simulink model "Klausur_fi_wi_ma"  (R2021b)
settings: Solver=FixedStepAuto  StartTime=0.0  StopTime=753.0  FixedStep=0,5  RelTol=1e-3
values from neighbouring files (symbols this model uses):
  A = 2.5    [untitled.m]
  cw = 0.4    [untitled.m]
  d = 0.6    [untitled.m]
  g = 9.81    [untitled.m]
  Height = load("Hoehe.txt")    [untitled.m]
  i1 = 12.5    [untitled.m]
  i2 = 5    [untitled.m]
  m = 2000    [untitled.m]
  max_torque = xlsread("Motorkennlinie.xlsx","C16:O16")    [untitled.m]
  p = 1.2    [untitled.m]
  RPM = out.RPM    [untitled.m]
  Time = load("Zeit.txt")    [untitled.m]
  Velocity = load("Geschwindigkeit.txt")    [untitled.m]
undefined symbols (not defined in the file or in its folder): f_roll, J, n
settings Model: Creator=under  LastModifiedBy=user

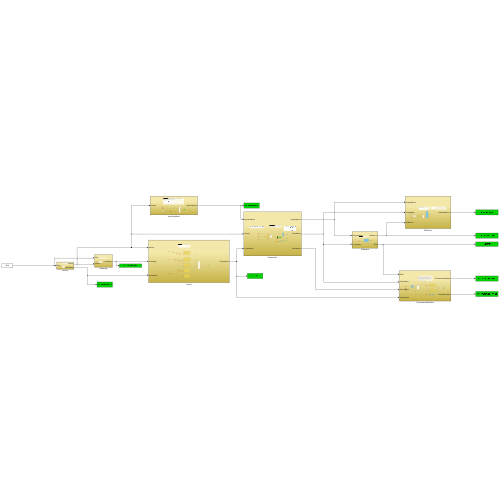
[thumbnail: Simulink's stored preview of the top-level diagram]
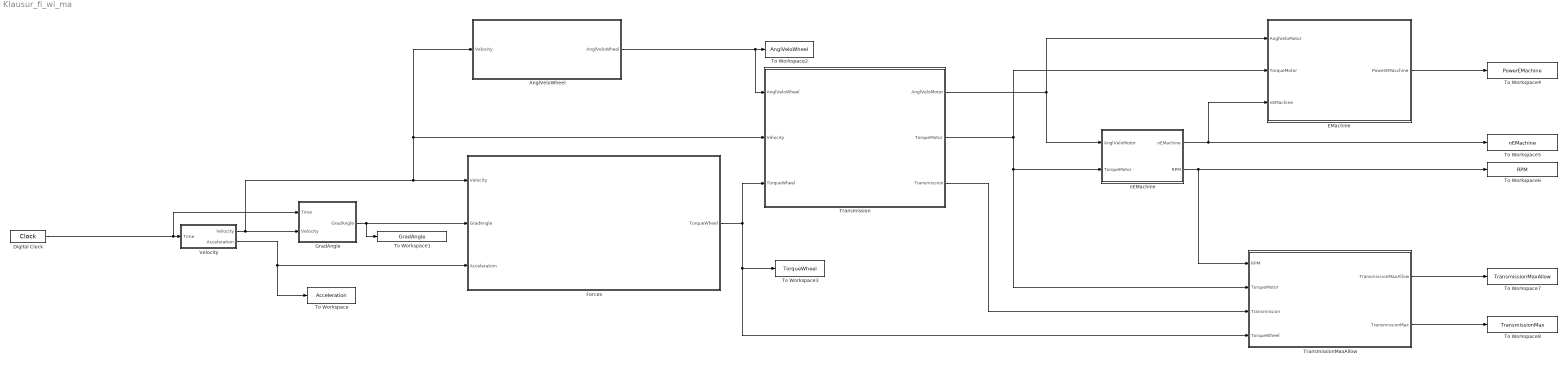
== system Klausur_fi_wi_ma ==
  AnglVeloWheel : Subsystem
  Digital Clock : DigitalClock
  EMachine : Subsystem
  Forces : Subsystem
  GradAngle : Subsystem
  To Workspace : ToWorkspace  VariableName=Acceleration  SaveFormat=Timeseries  SampleTime=-1
  To Workspace1 : ToWorkspace  VariableName=GradAngle  SaveFormat=Timeseries  SampleTime=-1
  To Workspace2 : ToWorkspace  VariableName=AnglVeloWheel  SaveFormat=Timeseries  SampleTime=-1
  To Workspace3 : ToWorkspace  VariableName=TorqueWheel  SaveFormat=Timeseries  SampleTime=-1
  To Workspace4 : ToWorkspace  VariableName=PowerEMachine  SaveFormat=Timeseries  SampleTime=-1
  To Workspace5 : ToWorkspace  VariableName=nEMachine  SaveFormat=Timeseries  SampleTime=-1
  To Workspace6 : ToWorkspace  VariableName=RPM  SaveFormat=Timeseries  SampleTime=-1
  To Workspace7 : ToWorkspace  VariableName=TransmissionMaxAllow  SaveFormat=Timeseries  SampleTime=-1
  To Workspace8 : ToWorkspace  VariableName=TransmissionMax  SaveFormat=Timeseries  SampleTime=-1
  Transmission : Subsystem
  TransmissionMaxAllow : Subsystem
  Velocity : Subsystem
  nEMachine : Subsystem
  wires:
  Transmission/2(TorqueMotor) -> TransmissionMaxAllow/2(TorqueMotor), nEMachine/2(TorqueMotor), EMachine/2(TorqueMotor)
  GradAngle/1(GradAngle) -> To Workspace1/1, Forces/2(GradAngle)
  Forces/1(TorqueWheel) -> TransmissionMaxAllow/4(TorqueWheel), To Workspace3/1, Transmission/3(TorqueWheel)
  Velocity/1(Velocity) -> AnglVeloWheel/1(Velocity), Transmission/2(Velocity), Forces/1(Velocity), GradAngle/2(Velocity)
  Digital Clock/1 -> GradAngle/1(Time), Velocity/1(Time)
  Transmission/1(AnglVeloMotor) -> EMachine/1(AnglVeloMotor), nEMachine/1(AnglVeloMotor)
  Velocity/2(Acceleration) -> To Workspace/1, Forces/3(Acceleration)
  AnglVeloWheel/1(AnglVeloWheel) -> Transmission/1(AnglVeloWheel), To Workspace2/1
  nEMachine/1(nEMachine) -> EMachine/3(nEMachine), To Workspace5/1
  EMachine/1(PowerEMaschine) -> To Workspace4/1
  nEMachine/2(RPM) -> TransmissionMaxAllow/1(RPM), To Workspace6/1
  Transmission/3(Transmission) -> TransmissionMaxAllow/3(Transmission)
  TransmissionMaxAllow/1(TransmissionMaxAllow) -> To Workspace7/1
  TransmissionMaxAllow/2(TransmissionMax) -> To Workspace8/1

== system Klausur_fi_wi_ma/AnglVeloWheel ==
  note: AnglVeloWheel
      | In diesem Subsystem wird die Geschwindigkeit und der Reifenradius dividiert, so wird die Winkelgeschwindigkeit ausgerechnet.
  Velocity : Inport
  Divide : Product  Inputs=*/
  WheelDiam : Constant  Value=d
  dToR : Gain  Gain=1/2
  AnglVeloWheel : Outport
  wires:
  dToR/1 -> Divide/2
  Velocity/1 -> Divide/1
  Divide/1 -> AnglVeloWheel/1
  WheelDiam/1 -> dToR/1

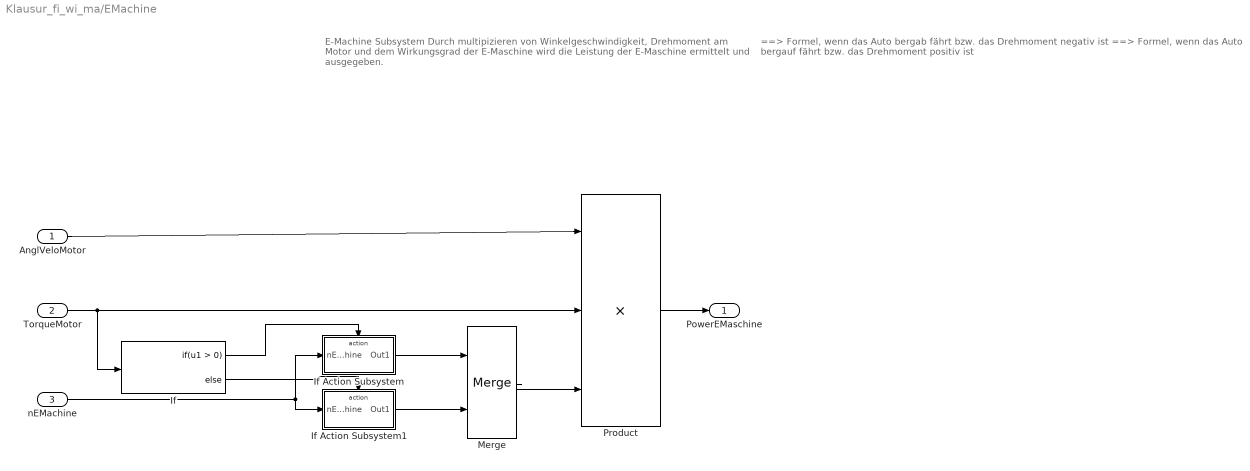
== system Klausur_fi_wi_ma/EMachine ==
  note: ==> Formel, wenn das Auto bergab fährt bzw. das Drehmoment negativ ist
      | ==> Formel, wenn das Auto bergauf fährt bzw. das Drehmoment positiv ist
  note: E-Machine Subsystem
      | Durch multipizieren von Winkelgeschwindigkeit, Drehmoment am Motor und dem Wirkungsgrad der E-Maschine wird die Leistung der E-Maschine ermittelt und ausgegeben.
  AnglVeloMotor : Inport
  TorqueMotor : Inport  Port=2
  nEMachine : Inport  Port=3
  If : If
  If Action Subsystem : Subsystem  TreatAsAtomicUnit=on
  If Action Subsystem1 : Subsystem  TreatAsAtomicUnit=on
  Merge : Merge
  Product : Product  Inputs=3
  PowerEMaschine : Outport
  wires:
  TorqueMotor/1 -> If/1, Product/2
  nEMachine/1 -> If Action Subsystem1/1(nEMachine), If Action Subsystem/1(nEMachine)
  If/2 -> If Action Subsystem1/Action
  If/1 -> If Action Subsystem/Action
  Product/1 -> PowerEMaschine/1
  Merge/1 -> Product/3
  If Action Subsystem/1(Out1) -> Merge/1
  If Action Subsystem1/1(Out1) -> Merge/2
  AnglVeloMotor/1 -> Product/1

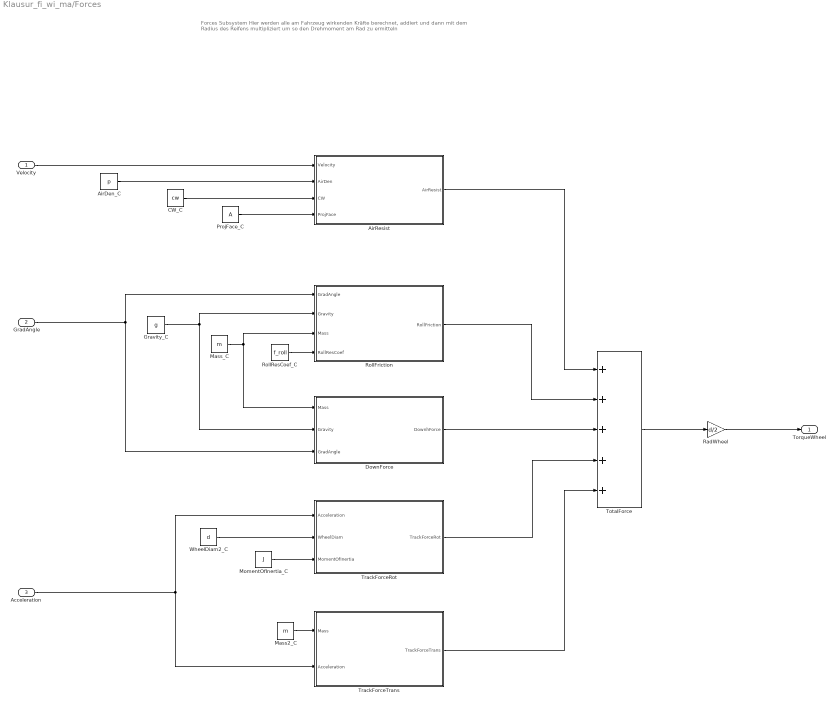
== system Klausur_fi_wi_ma/Forces ==
  note: Forces Subsystem
      | Hier werden alle am Fahrzeug wirkenden Kräfte berechnet, addiert und dann mit dem Radius des Reifens multipliziert um so den Drehmoment am Rad zu ermitteln
  Velocity : Inport
  GradAngle : Inport  Port=2
  Acceleration : Inport  Port=3
  AirDen_C : Constant  Value=p
  AirResist : Subsystem
  CW_C : Constant  Value=cw
  DownForce : Subsystem
  Gravity_C : Constant  Value=g
  Mass2_C : Constant  Value=m
  Mass_C : Constant  Value=m
  MomentOfInertia_C : Constant  Value=J
  ProjFace_C : Constant  Value=A
  RadWheel : Gain  Gain=d/2
  RollFriction : Subsystem
  RollResCoef_C : Constant  Value=f_roll
  TotalForce : Sum  Inputs=+++++
  TrackForceRot : Subsystem
  TrackForceTrans : Subsystem
  WheelDiam2_C : Constant  Value=d
  TorqueWheel : Outport
  wires:
  GradAngle/1 -> DownForce/3(GradAngle), RollFriction/1(GradAngle)
  Gravity_C/1 -> DownForce/2(Gravity), RollFriction/2(Gravity)
  RollResCoef_C/1 -> RollFriction/4(RollResCoef)
  Mass_C/1 -> DownForce/1(Mass), RollFriction/3(Mass)
  TotalForce/1 -> RadWheel/1
  Acceleration/1 -> TrackForceTrans/2(Acceleration), TrackForceRot/1(Acceleration)
  TrackForceRot/1(TrackForceRot) -> TotalForce/4
  TrackForceTrans/1(TrackForceTrans) -> TotalForce/5
  WheelDiam2_C/1 -> TrackForceRot/2(WheelDiam)
  MomentOfInertia_C/1 -> TrackForceRot/3(MomentOfInertia)
  Mass2_C/1 -> TrackForceTrans/1(Mass)
  RadWheel/1 -> TorqueWheel/1
  AirResist/1(AirResist) -> TotalForce/1
  Velocity/1 -> AirResist/1(Velocity)
  ProjFace_C/1 -> AirResist/4(ProjFace)
  CW_C/1 -> AirResist/3(CW)
  AirDen_C/1 -> AirResist/2(AirDen)
  RollFriction/1(RollFriction) -> TotalForce/2
  DownForce/1(DownhForce) -> TotalForce/3

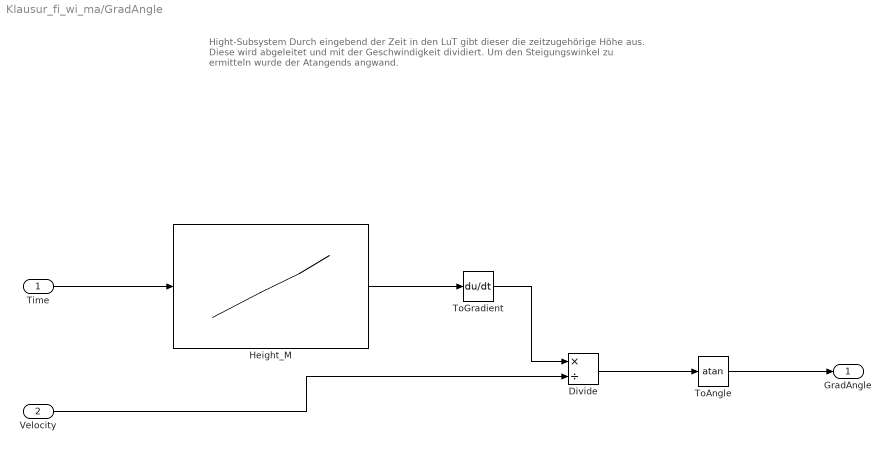
== system Klausur_fi_wi_ma/GradAngle ==
  note: Hight-Subsystem
      | Durch eingebend der Zeit in den LuT gibt dieser die zeitzugehörige Höhe aus. Diese wird abgeleitet und mit der Geschwindigkeit dividiert. Um den Steigungswinkel zu ermitteln wurde der Atangends angwand.
  Time : Inport
  Velocity : Inport  Port=2
  Divide : Product  Inputs=*/
  Height_M : Lookup_n-D  NumberOfTableDimensions=1  BreakpointsForDimension1=Time  Table=Height  InternalRulePriority=Speed  RndMeth=Simplest  InputSameDT=on
  ToAngle : Trigonometry  Operator=atan
  ToGradient : Derivative
  GradAngle : Outport
  wires:
  ToAngle/1 -> GradAngle/1
  Divide/1 -> ToAngle/1
  Velocity/1 -> Divide/2
  ToGradient/1 -> Divide/1
  Height_M/1 -> ToGradient/1
  Time/1 -> Height_M/1

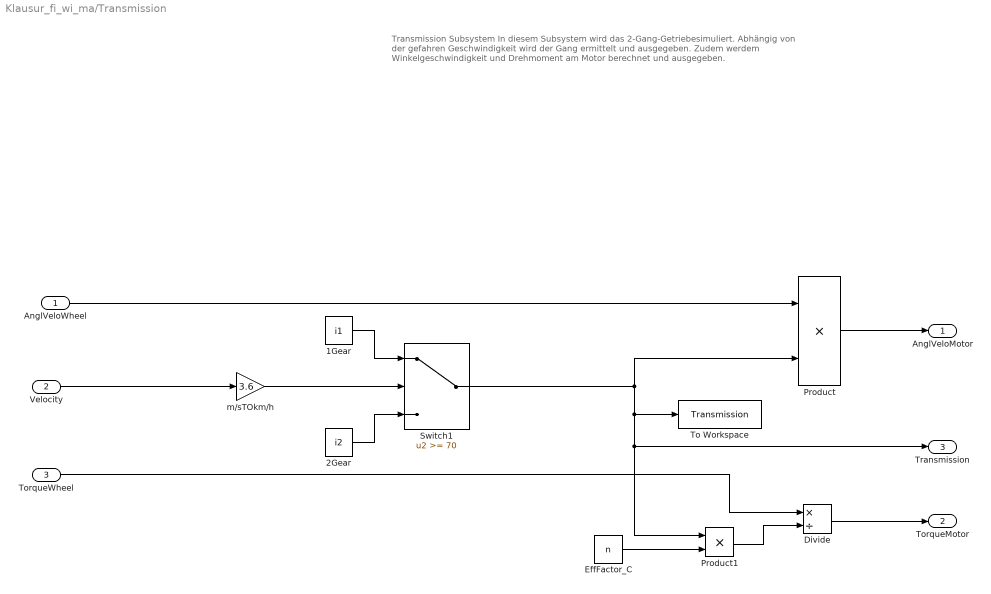
== system Klausur_fi_wi_ma/Transmission ==
  note: Transmission Subsystem
      | In diesem Subsystem wird das 2-Gang-Getriebesimuliert. Abhängig von der gefahren Geschwindigkeit wird der Gang ermittelt und ausgegeben.
      | Zudem werdem Winkelgeschwindigkeit und Drehmoment am Motor berechnet und ausgegeben.
  AnglVeloWheel : Inport
  Velocity : Inport  Port=2
  TorqueWheel : Inport  Port=3
  1Gear : Constant  Value=i1
  2Gear : Constant  Value=i2
  Divide : Product  Inputs=*/
  EffFactor_C : Constant  Value=n
  Product : Product
  Product1 : Product
  Switch1 : Switch  Threshold=70
  To Workspace : ToWorkspace  VariableName=Transmission  SaveFormat=Timeseries  SampleTime=-1
  "m/sTOkm/h  " : Gain  Gain=3.6
  AnglVeloMotor : Outport
  TorqueMotor : Outport  Port=2
  Transmission : Outport  Port=3
  wires:
  "m/sTOkm/h  "/1 -> Switch1/2
  Switch1/1 -> Transmission/1, Product1/1, To Workspace/1, Product/2
  Product/1 -> AnglVeloMotor/1
  EffFactor_C/1 -> Product1/2
  Product1/1 -> Divide/2
  TorqueWheel/1 -> Divide/1
  Divide/1 -> TorqueMotor/1
  Velocity/1 -> "m/sTOkm/h  "/1
  AnglVeloWheel/1 -> Product/1
  1Gear/1 -> Switch1/1
  2Gear/1 -> Switch1/3

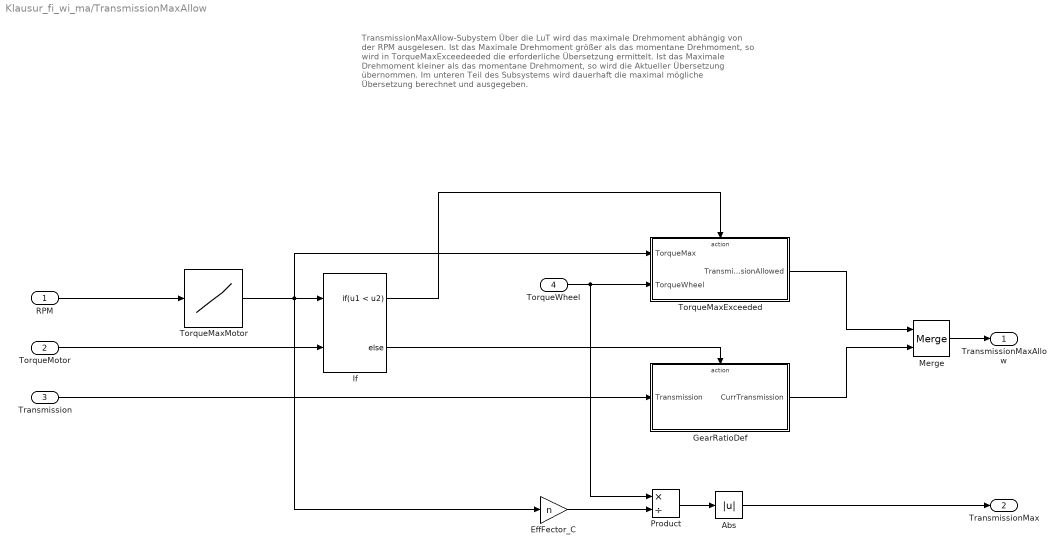
== system Klausur_fi_wi_ma/TransmissionMaxAllow ==
  note: TransmissionMaxAllow-Subystem
      | Über die LuT wird das maximale Drehmoment abhängig von der RPM ausgelesen. Ist das Maximale Drehmoment größer als das momentane Drehmoment, so wird in TorqueMaxExceedeeded die erforderliche Übersetzung ermittelt. Ist das Maximale Drehmoment kleiner als das momentane Drehmoment, so wird die Aktueller Übersetzung übernommen.
      | Im unteren Teil des Subsystems wird dauerhaft die maximal mögliche Übersetzung berechnet und ausgegeben.
  RPM : Inport
  TorqueMotor : Inport  Port=2
  Transmission : Inport  Port=3
  TorqueWheel : Inport  Port=4
  Abs : Abs
  EffFector_C : Gain  Gain=n
  GearRatioDef : Subsystem  TreatAsAtomicUnit=on
  If : If  NumInputs=2  IfExpression=u1 < u2
  Merge : Merge
  Product : Product  Inputs=*/
  TorqueMaxExceeded : Subsystem  TreatAsAtomicUnit=on
  TorqueMaxMotor : Lookup_n-D  NumberOfTableDimensions=1  BreakpointsForDimension1=RPM  Table=max_torque  InternalRulePriority=Speed  RndMeth=Simplest  InputSameDT=on
  TransmissionMaxAllow : Outport
  TransmissionMax : Outport  Port=2
  wires:
  Abs/1 -> TransmissionMax/1
  TorqueMaxMotor/1 -> EffFector_C/1, If/1, TorqueMaxExceeded/1(TorqueMax)
  If/1 -> TorqueMaxExceeded/Action
  TorqueWheel/1 -> Product/1, TorqueMaxExceeded/2(TorqueWheel)
  EffFector_C/1 -> Product/2
  Product/1 -> Abs/1
  TorqueMaxExceeded/1(TransmissionAllowed) -> Merge/1
  GearRatioDef/1(CurrTransmission) -> Merge/2
  RPM/1 -> TorqueMaxMotor/1
  TorqueMotor/1 -> If/2
  If/2 -> GearRatioDef/Action
  Transmission/1 -> GearRatioDef/1(Transmission)
  Merge/1 -> TransmissionMaxAllow/1

== system Klausur_fi_wi_ma/Velocity ==
  note: Velocity-Subsystem
      | Durch die Zeit werden die passenden Werte der Geschwindigkeit aus dem LuT in das System gegeben. Um die Beschleunigung zu berechen wurde die Geschwindigkeit abgeleitet.
  Time : Inport
  Velocity_M : Lookup_n-D  NumberOfTableDimensions=1  BreakpointsForDimension1=Time  Table=Velocity  InternalRulePriority=Speed  RndMeth=Simplest  InputSameDT=on
  VtoA : Derivative
  Velocity : Outport
  Acceleration : Outport  Port=2
  wires:
  VtoA/1 -> Acceleration/1
  Time/1 -> Velocity_M/1
  Velocity_M/1 -> Velocity/1, VtoA/1  "Speed"

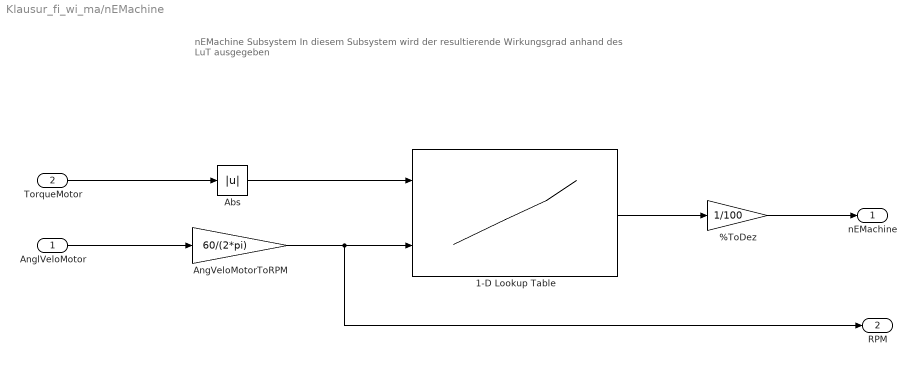
== system Klausur_fi_wi_ma/nEMachine ==
  note: nEMachine Subsystem
      | In diesem Subsystem wird der resultierende Wirkungsgrad anhand des LuT ausgegeben
  AnglVeloMotor : Inport
  TorqueMotor : Inport  Port=2
  %ToDez : Gain  Gain=1/100
  1-D Lookup Table : Lookup_n-D  BreakpointsForDimension1=|  BreakpointsForDimension2="[0\t1000\t2000\t3000\t4000\t5000\t6000\t7000\t8000\t9000\t10000\t11000\t12000]"  Table=|  InternalRulePriority=Speed  RndMeth=Simplest  InputSameDT=on
      BreakpointsForDimension1=|
      | [0
      | 25
      | 50
      | 75
      | 100
      | 125
      | 150
      | 175
      | 200
      | 225
      | 250]
      Table=|
      | [50	61	70	74	78	76	73	73	69	68	68	67	65
      | 64	75	85	85	86	87	88	90	88	87	87	86	86
      | 70	81	87	89	91	92	93	93	94	93	91	91	92
      | 69	81	88	89	91	92	93	94	94	94	93	93	91
      | 68	79	87	91	92	93	94	94	93	93	92	92	91
      | 68	79	87	90	92	93	94	94	92	92	92	92	91
      | 66	78	87	90	92	93	93	93	92	92	92	92	91
      | 65	78	86	90	91	93	93	93	92	92	92	92	91
      | 63	77	86	89	91	92	93	93	92	92	92	91	91
      | 62	76	85	88	91	92	92	92	92	91	91	91	91
      | 60	75	84	88	90	91	91	91	91	91	91	91	91]
      settings: InputPortMap=u0,u1
  Abs : Abs
  AngVeloMotorToRPM : Gain  Gain=60/(2*pi)
  nEMachine : Outport
  RPM : Outport  Port=2
  wires:
  TorqueMotor/1 -> Abs/1
  %ToDez/1 -> nEMachine/1
  1-D Lookup Table/1 -> %ToDez/1
  Abs/1 -> 1-D Lookup Table/1
  AngVeloMotorToRPM/1 -> RPM/1, 1-D Lookup Table/2
  AnglVeloMotor/1 -> AngVeloMotorToRPM/1

== system Klausur_fi_wi_ma/EMachine/If Action Subsystem ==
  nEMachine : Inport
  Action Port : ActionPort  ActionPortLabel=if(u1 > 0)
  Constant : Constant
  Divide : Product  Inputs=*/
  Out1 : Outport
  wires:
  nEMachine/1 -> Divide/2
  Constant/1 -> Divide/1
  Divide/1 -> Out1/1

== system Klausur_fi_wi_ma/EMachine/If Action Subsystem1 ==
  nEMachine : Inport
  Action Port : ActionPort  ActionPortLabel=else
  Out1 : Outport
  wires:
  nEMachine/1 -> Out1/1

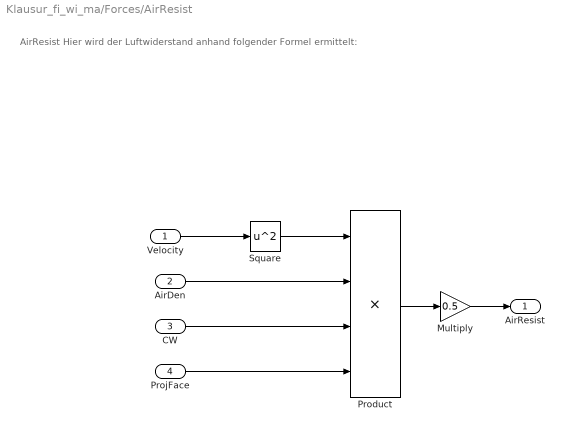
== system Klausur_fi_wi_ma/Forces/AirResist ==
  note: AirResist
      | Hier wird der Luftwiderstand anhand folgender Formel ermittelt:
  Velocity : Inport
  AirDen : Inport  Port=2
  CW : Inport  Port=3
  ProjFace : Inport  Port=4
  Multiply : Gain  Gain=0.5
  Product : Product  Inputs=4
  Square : Math  Operator=square  SaturateOnIntegerOverflow=on
  AirResist : Outport
  wires:
  ProjFace/1 -> Product/4
  Velocity/1 -> Square/1
  CW/1 -> Product/3
  Product/1 -> Multiply/1
  Square/1 -> Product/1
  AirDen/1 -> Product/2
  Multiply/1 -> AirResist/1

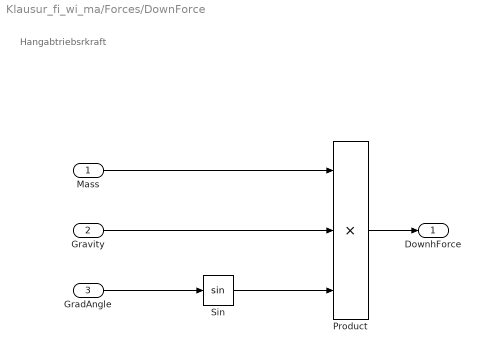
== system Klausur_fi_wi_ma/Forces/DownForce ==
  note: Hangabtriebsrkraft
  Mass : Inport
  Gravity : Inport  Port=2
  GradAngle : Inport  Port=3
  Product : Product  Inputs=3
  Sin : Trigonometry
  DownhForce : Outport
  wires:
  Gravity/1 -> Product/2
  GradAngle/1 -> Sin/1
  Product/1 -> DownhForce/1
  Sin/1 -> Product/3
  Mass/1 -> Product/1

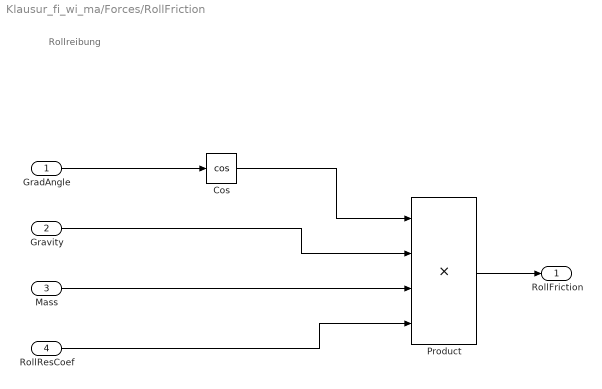
== system Klausur_fi_wi_ma/Forces/RollFriction ==
  note: Rollreibung
  GradAngle : Inport
  Gravity : Inport  Port=2
  Mass : Inport  Port=3
  RollResCoef : Inport  Port=4
  Cos : Trigonometry  Operator=cos
  Product : Product  Inputs=4
  RollFriction : Outport
  wires:
  Product/1 -> RollFriction/1
  GradAngle/1 -> Cos/1
  Cos/1 -> Product/1
  Gravity/1 -> Product/2
  Mass/1 -> Product/3
  RollResCoef/1 -> Product/4

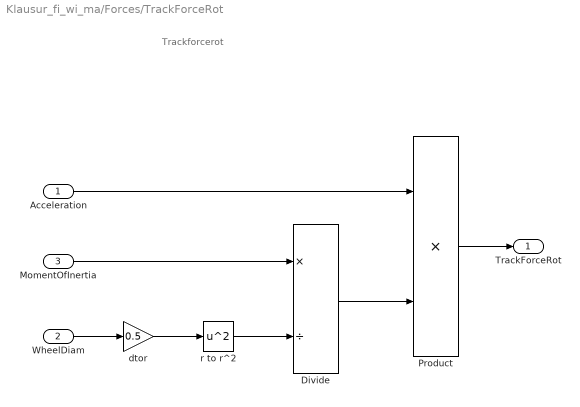
== system Klausur_fi_wi_ma/Forces/TrackForceRot ==
  note: Trackforcerot
  Acceleration : Inport
  WheelDiam : Inport  Port=2
  MomentOfInertia : Inport  Port=3
  Divide : Product  Inputs=*/
  Product : Product
  dtor : Gain  Gain=0.5
  r to r^2 : Math  Operator=square  SaturateOnIntegerOverflow=on
  TrackForceRot : Outport
  wires:
  WheelDiam/1 -> dtor/1
  MomentOfInertia/1 -> Divide/1
  dtor/1 -> r to r^2/1
  r to r^2/1 -> Divide/2
  Divide/1 -> Product/2
  Acceleration/1 -> Product/1
  Product/1 -> TrackForceRot/1

== system Klausur_fi_wi_ma/Forces/TrackForceTrans ==
  note: Trackforcetrans
  Mass : Inport
  Acceleration : Inport  Port=2
  Product : Product
  TrackForceTrans : Outport
  wires:
  Mass/1 -> Product/1
  Acceleration/1 -> Product/2
  Product/1 -> TrackForceTrans/1

== system Klausur_fi_wi_ma/TransmissionMaxAllow/GearRatioDef ==
  Transmission : Inport
  Action Port : ActionPort  ActionPortLabel=else
  CurrTransmission : Outport
  wires:
  Transmission/1 -> CurrTransmission/1

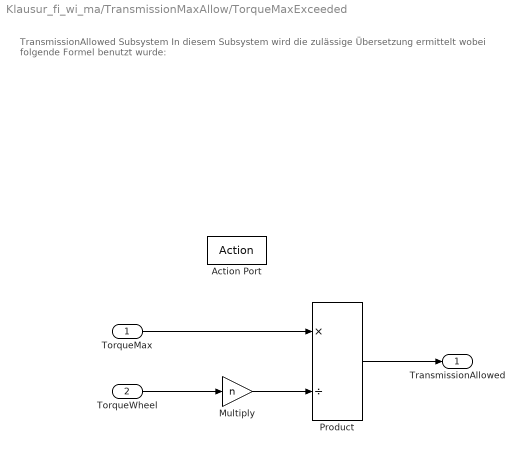
== system Klausur_fi_wi_ma/TransmissionMaxAllow/TorqueMaxExceeded ==
  note: TransmissionAllowed Subsystem
      | In diesem Subsystem wird die zulässige Übersetzung ermittelt wobei folgende Formel benutzt wurde:
  TorqueMax : Inport
  TorqueWheel : Inport  Port=2
  Action Port : ActionPort  ActionPortLabel=if(u1 < u2)
  Multiply : Gain  Gain=n
  Product : Product  Inputs=*/
  TransmissionAllowed : Outport
  wires:
  TorqueMax/1 -> Product/1
  Multiply/1 -> Product/2
  TorqueWheel/1 -> Multiply/1
  Product/1 -> TransmissionAllowed/1
